simulink model "PV_Inverter"  (R2018b)
settings: Solver=ode45  StartTime=0*24*3600  StopTime=3600  MaxStep=60  RelTol=1e-4  EnableMultiTasking=on
undefined symbols (not defined in the file): path_carnot, phase
libraries: carnot x2, simulink x1
settings Model: Creator=drhf  LastModifiedBy=drhf
settings DataIOCC: LimitDataPoints=on  SaveFormat=Array  SignalLoggingSaveFormat=ModelDataLogs
settings OptimizationCC: ExpressionDepthLimit=2147483647  LifeSpan=inf
settings DebuggingCC: UnderspecifiedInitializationDetection=Classic  MergeDetectMultiDrivingBlocksExec=none  SolverPrmCheckMsg=warning  FcnCallInpInsideContextMsg=warning  StateNameClashWarn=warning  SFUnexpectedBacktrackingDiag=warning  SFNoUnconditionalDefaultTransitionDiag=warning  SFExecutionAtInitializationDiag=none
settings HardwareCC: ProdBitPerPointer=32  ProdBitPerSizeT=32  ProdBitPerPtrDiffT=32  ProdLargestAtomicFloat=None  ProdIntDivRoundTo=Undefined  ProdEndianess=Unspecified  ProdWordSize=32  ProdHWDeviceType=32-bit Generic
settings ModelReferenceCC: PropagateSignalLabelsOutOfModel=off
settings SFSimCC: SimUseLocalCustomCode=off
settings RTWCC: RTWUseLocalCustomCode=off
settings CodeAppCC: StateflowObjectComments=on
settings GRTTargetCC: TargetLangStandard=C89/C90 (ANSI)  GeneratePreprocessorConditionals=Disable all  CombineOutputUpdateFcns=off  GRTInterface=on
settings ConfigComp: CovMetricSettings=dw  CovHtmlReporting=on  CovSaveCumulativeToWorkspaceVar=on  CovSaveSingleToWorkspaceVar=on  CovExternalEMLEnable=off

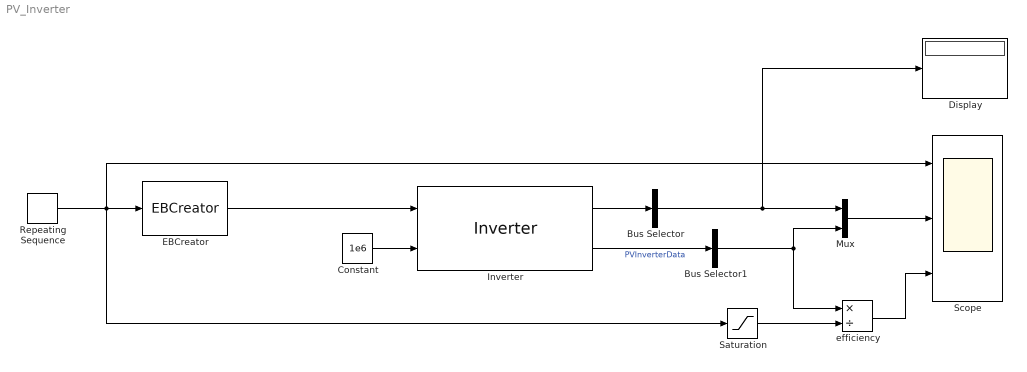
== system PV_Inverter ==
  Bus Selector : BusSelector  OutputSignals=ActPower1,ActPower2,ActPower3  OutputAsBus=on
  Bus Selector1 : BusSelector  OutputSignals=P_AC  OutputAsBus=on
  Constant : Constant  Value=1e6
  Display : Display
  EBCreator : carnot/Basic/Electric/EBCreator  Inport_ID=off  Inport_f=off  Inport_v1=off  Inport_p1=on  Inport_pf1=off  Inport_v2=off  Inport_p2=off  Inport_pf2=off  Inport_v3=off  Inport_p3=off  Inport_pf3=off  ID=20001  f=20  v1=0  p1=1e5  pf1=1  v2=0  p2=1e5  pf2=1  v3=0  p3=1e5  pf3=1  Annotation_ID=off  Annotation_f=off  Annotation_v1=off  Annotation_p1=off  Annotation_pf1=off  Annotation_v2=off  Annotation_p2=off  Annotation_pf2=off  Annotation_v3=off  Annotation_p3=off  Annotation_pf3=on
      settings: AttributesFormatString=1 power factor
  Inverter : carnot/Source/Electric_Generator/Inverter  PathName=fullfile(path_carnot('libsl'), 'Source', 'Electric_Generator', 'Inverter', 'parameter_set')  FileName='SMA_SB1_5_VL40.mat'  userPath=off  userParam=off  Pacnom=1500  nphase=1-phase  U=230  f=50  PstepsEta=[0 0.1 0.2 0.25 0.3 0.5 0.75 1]  Eta=[0 0.927 0.955 0.96 0.964 0.97 0.972 0.972]  P_standby=1
  Mux : Mux  Inputs=2
  Repeating Sequence : simulink/Sources/Repeating Sequence  rep_seq_t=[0 10 3600 4000]  rep_seq_y=[0 0 1 1]*20e3
  Saturation : Saturate  UpperLimit=inf  LowerLimit=100
  Scope : Scope  NumInputPorts=3
  efficiency : Product  Inputs=*/
  wires:
  Repeating Sequence/1 -> Scope/1, Saturation/1, EBCreator/1
  Inverter/1 -> Bus Selector/1
  efficiency/1 -> Scope/3
  Saturation/1 -> efficiency/2
  Constant/1 -> Inverter/2
  Inverter/2 -> Bus Selector1/1  "PVInverterData"
  Bus Selector/1 -> Display/1, Mux/1
  EBCreator/1 -> Inverter/1
  Bus Selector1/1 -> Mux/2, efficiency/1
  Mux/1 -> Scope/2
